simulink model "H1"  (R2023b)
settings: Solver=FixedStepAuto  StartTime=0.0  StopTime=inf  RelTol=1e-3  EnableMultiTasking=on
libraries: simulink x8
settings Model: ExtModeTrigDuration=2  Creator=Carlos  LastModifiedBy=adria
settings SolverCC: AutoInsertRateTranBlk=on
settings OptimizationCC: EnhancedBackFolding=on  PassReuseOutputArgsAs=Individual arguments  ZeroExternalMemoryAtStartup=off  ZeroInternalMemoryAtStartup=off  MaxStackSize=64  OptimizeBlockOrder=speed  DifferentSizesBufferReuse=on  OptimizationCustomize=off  EfficientTunableParamExpr=on
settings DebuggingCC: ParameterTunabilityLossMsg=error
settings HardwareCC: ProdBitPerInt=16  ProdBitPerPointer=16  ProdBitPerSizeT=16  ProdBitPerPtrDiffT=16  ProdLargestAtomicFloat=None  ProdWordSize=8  ProdHWDeviceType=Atmel->AVR  UseEmbeddedCoderFeatures=off  UseSimulinkCoderFeatures=off
settings SFSimCC: MATLABDynamicMemAlloc=off
settings RTWCC: Description=Embedded Coder  SystemTargetFile=ert.tlc  HardwareBoard=Arduino Mega 2560  TemplateMakefile=ert_default_tmf  Toolchain=Arduino AVR  BuildConfiguration=Faster Runs
settings CodeAppCC: ForceParamTrailComments=on  IgnoreCustomStorageClasses=off  OperatorAnnotations=on  SimulinkDataObjDesc=on  SFDataObjDesc=on  MangleLength=10  InsertBlockDesc=on
settings ERTTargetCC: SupportContinuousTime=on  SupportNonInlinedSFcns=on  SupportVariableSizeSignals=on  ExtModeTransport=3  ExtModeStaticAlloc=on  ExtModeAutomaticAllocSize=off  ExtModeStaticAllocSize=2048  ExtModeMexFile=ext_xcp  ExtModeIntrfLevel=Level2 - Open

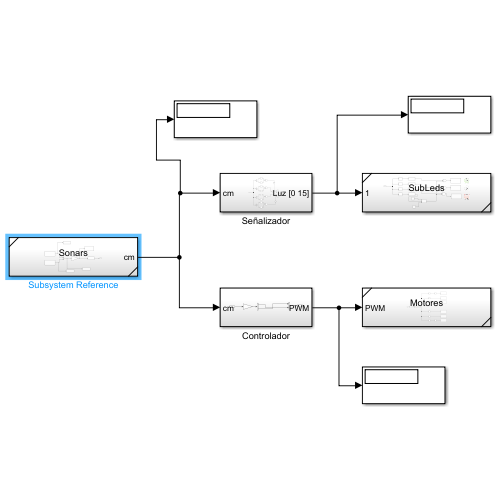
[thumbnail: Simulink's stored preview of the top-level diagram]
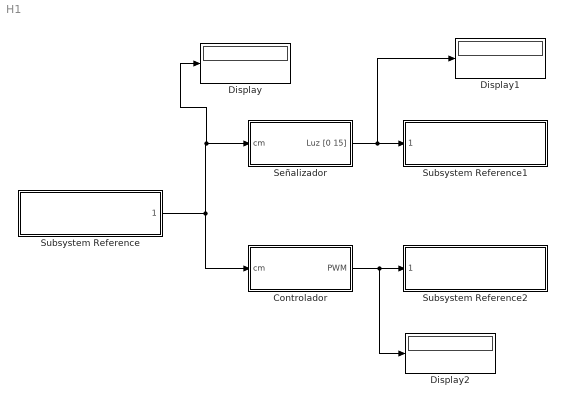
== system H1 ==
  Controlador : Subsystem
  Display : Display
  Display1 : Display
  Display2 : Display
  Señalizador : Subsystem
  Subsystem Reference : Subsystem  ReferencedSubsystem=Sonars
  Subsystem Reference1 : Subsystem  ReferencedSubsystem=SubLeds
  Subsystem Reference2 : Subsystem  ReferencedSubsystem=Motores
  wires:
  Subsystem Reference/1 -> Display/1, Señalizador/1(cm), Controlador/1(cm)
  Controlador/1(PWM) -> Display2/1, Subsystem Reference2/1
  Señalizador/1(Luz [0 15]) -> Display1/1, Subsystem Reference1/1

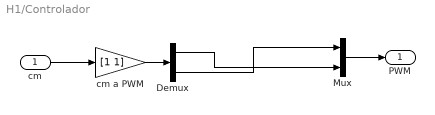
== system H1/Controlador ==
  cm : Inport  OutDataTypeStr=int16
  Demux : Demux  Outputs=2
  Mux : Mux  Inputs=2
  cm a PWM : Gain  Gain=[1 1]  ParamDataTypeStr=int16  OutDataTypeStr=int16
  PWM : Outport  OutDataTypeStr=int16
  wires:
  Mux/1 -> PWM/1
  cm/1 -> cm a PWM/1
  Demux/2 -> Mux/1
  Demux/1 -> Mux/2
  cm a PWM/1 -> Demux/1

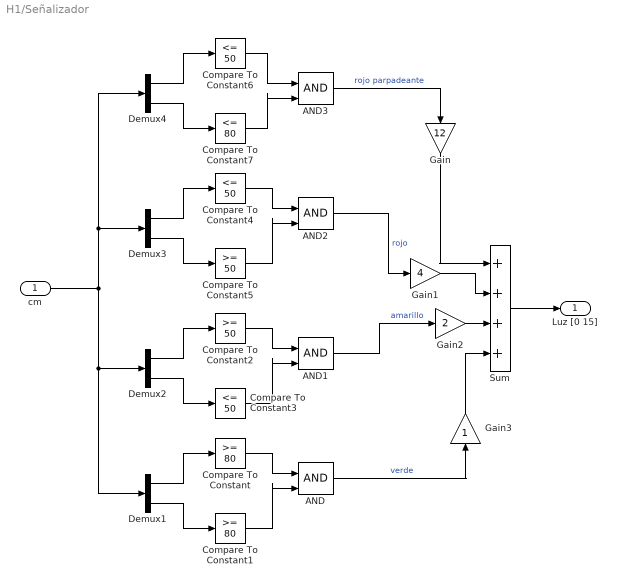
== system H1/Señalizador ==
  cm : Inport  OutDataTypeStr=int16
  AND{,1..3} (4 alike) : Logic  IconShape=distinctive  AllPortsSameDT=off  OutDataTypeStr=boolean
  Compare To Constant : simulink/Logic and Bit Operations/Compare To Constant  relop=>=  const=80  OutDataTypeStr=boolean
  Compare To Constant1 : simulink/Logic and Bit Operations/Compare To Constant  relop=>=  const=80  OutDataTypeStr=boolean
  Compare To Constant2 : simulink/Logic and Bit Operations/Compare To Constant  relop=>=  const=50  OutDataTypeStr=boolean
  Compare To Constant3 : simulink/Logic and Bit Operations/Compare To Constant  relop=<=  const=50  OutDataTypeStr=boolean
  Compare To Constant4 : simulink/Logic and Bit Operations/Compare To Constant  relop=<=  const=50  OutDataTypeStr=boolean
  Compare To Constant5 : simulink/Logic and Bit Operations/Compare To Constant  relop=>=  const=50  OutDataTypeStr=boolean
  Compare To Constant6 : simulink/Logic and Bit Operations/Compare To Constant  relop=<=  const=50  OutDataTypeStr=boolean
  Compare To Constant7 : simulink/Logic and Bit Operations/Compare To Constant  relop=<=  const=80  OutDataTypeStr=boolean
  Demux{1..4} (4 alike) : Demux  Outputs=2
  Gain : Gain  Gain=12  ParamDataTypeStr=int16  OutDataTypeStr=int16
  Gain1 : Gain  Gain=4  ParamDataTypeStr=int16  OutDataTypeStr=int16
  Gain2 : Gain  Gain=2  ParamDataTypeStr=int16  OutDataTypeStr=int16
  Gain3 : Gain  ParamDataTypeStr=int16  OutDataTypeStr=int16
  Sum : Sum  Inputs=++++
  Luz [0 15] : Outport  OutDataTypeStr=int16
  wires:
  Demux1/2 -> Compare To Constant1/1
  Demux1/1 -> Compare To Constant/1
  Compare To Constant/1 -> AND/1
  Compare To Constant1/1 -> AND/2
  cm/1 -> Demux3/1, Demux4/1, Demux1/1, Demux2/1
  Compare To Constant3/1 -> AND1/2
  Demux2/2 -> Compare To Constant3/1
  Demux2/1 -> Compare To Constant2/1
  Compare To Constant2/1 -> AND1/1
  Compare To Constant4/1 -> AND2/1
  Demux3/1 -> Compare To Constant4/1
  Demux3/2 -> Compare To Constant5/1
  Compare To Constant5/1 -> AND2/2
  Demux4/1 -> Compare To Constant6/1
  Compare To Constant6/1 -> AND3/1
  Compare To Constant7/1 -> AND3/2
  Demux4/2 -> Compare To Constant7/1
  AND2/1 -> Gain1/1  "rojo"
  AND1/1 -> Gain2/1  "amarillo"
  AND/1 -> Gain3/1  "verde"
  Sum/1 -> Luz [0 15]/1
  AND3/1 -> Gain/1  "rojo parpadeante"
  Gain/1 -> Sum/1
  Gain1/1 -> Sum/2
  Gain2/1 -> Sum/3
  Gain3/1 -> Sum/4
